simulink model "APE_1"  (R2025a)
settings: Solver=VariableStepAuto  StartTime=0.0  StopTime=1.016  RelTol=1e-3
libraries: spsPWMGeneratorDCDCLib x8, spsCurrentMeasurementLib x5, spsMosfetLib x4, spsSeriesRLCBranchLib x4, spsVoltageMeasurementLib x3, spsDCVoltageSourceLib x1, spsGroundLib x1, eeStairGenerator x1, sps_lib x1
settings Model: Creator=KAILASH  LastModifiedBy=KAILASH

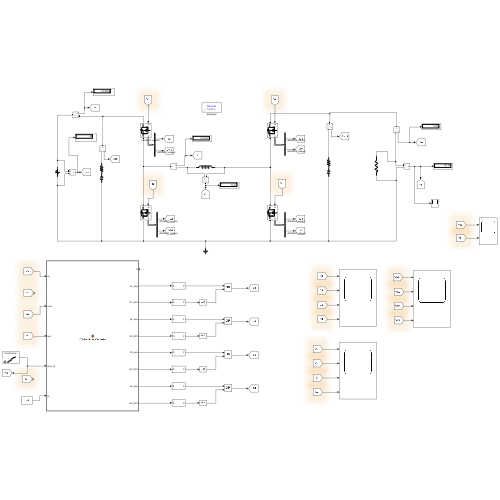
[thumbnail: Simulink's stored preview of the top-level diagram]
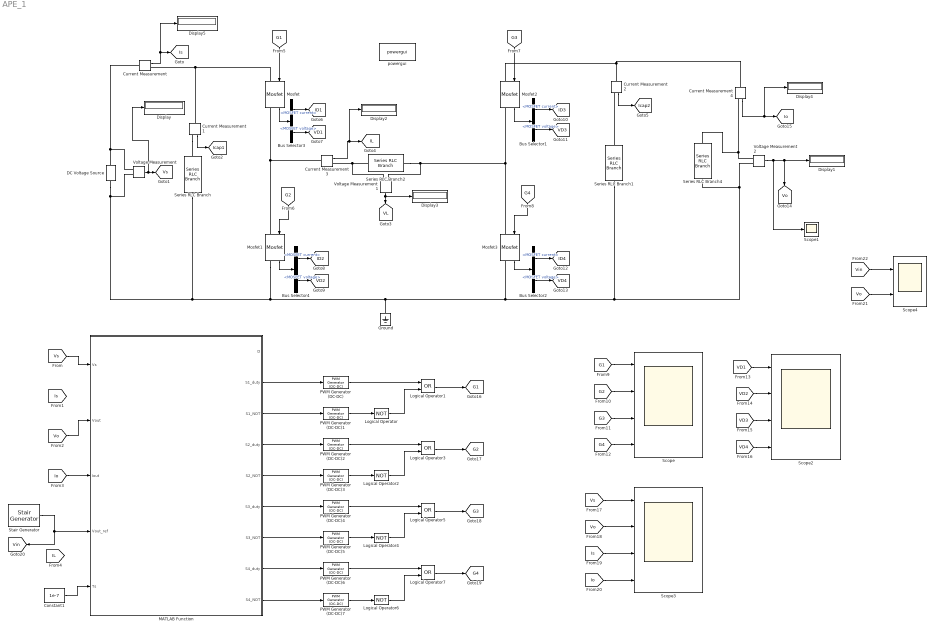
== system APE_1 ==
  Bus Selector{1..4} (4 alike) : BusSelector  OutputSignals=MOSFET current,MOSFET voltage
  Constant1 : Constant  Value=1e-7
  Current Measurement{,1..4} (5 alike) : spsCurrentMeasurementLib/Current Measurement  PhasorSimulation=off  OutputType=Complex  PSBequivalent=0
  DC Voltage Source : spsDCVoltageSourceLib/DC Voltage Source  Amplitude=48  Measurements=Voltage
  Display{,1..5} (6 alike) : Display
  Ground : spsGroundLib/Ground  LConnTagsString=a
  Logical Operator{,2,4,6} (4 alike) : Logic  Operator=NOT  AllPortsSameDT=off  OutDataTypeStr=boolean
  Logical Operator{1,3,5,7} (4 alike) : Logic  Operator=OR  AllPortsSameDT=off  OutDataTypeStr=boolean
  MATLAB Function : MATLAB Function  TreatAsAtomicUnit=on
  Mosfet{,1..3} (4 alike) : spsMosfetLib/Mosfet  Ron=0.01  Lon=0  Rd=0.01  Vfd=0.8  IC=0  Rs=1e5  Cs=inf  Measurements=on
  PWM Generator (DC-DC){,1..7} (8 alike) : spsPWMGeneratorDCDCLib/PWM Generator (DC-DC)  Fsw=75e3  Ts=1e-7
  Scope : Scope  NumInputPorts=4
      settings: ActiveDisplayYMinimum=0.9  ActiveDisplayYMaximum=1.1
  Scope1 : Scope
      settings: ActiveDisplayYMinimum=-11.04407431649155  ActiveDisplayYMaximum=99.45668137748801
  Scope2 : Scope  NumInputPorts=4
      settings: ActiveDisplayYMinimum=-4.0101855999563254  ActiveDisplayYMaximum=36.044750018114769  DataLoggingVariableName=ScopeData2
  Scope3 : Scope  NumInputPorts=4
      settings: ActiveDisplayYMinimum=38  ActiveDisplayYMaximum=58  DataLoggingVariableName=ScopeData3
  Scope4 : Scope  NumInputPorts=2
      settings: ActiveDisplayYMinimum=-26.842242201674949  ActiveDisplayYMaximum=241.58017981507462  DataLoggingVariableName=ScopeData4
  Series RLC Branch : spsSeriesRLCBranchLib/Series RLC Branch  LConnTagsString=__new0  RConnTagsString=__new0  BranchType=RC  Resistance=0.001  Inductance=1e-3  SetiL0=off  InitialCurrent=0  Capacitance=488e-6  Setx0=off  InitialVoltage=48  Measurements=None
  Series RLC Branch1 : spsSeriesRLCBranchLib/Series RLC Branch  LConnTagsString=__new0  RConnTagsString=__new0  BranchType=RC  Resistance=0.01  Inductance=1e-3  SetiL0=off  InitialCurrent=0  Capacitance=488e-6  Setx0=off  InitialVoltage=36  Measurements=None
  Series RLC Branch2 : spsSeriesRLCBranchLib/Series RLC Branch  LConnTagsString=__new0  RConnTagsString=__new0  BranchType=L  Resistance=1  Inductance=150e-6  SetiL0=off  InitialCurrent=0  Capacitance=1e-6  Setx0=off  InitialVoltage=0  Measurements=None
  Series RLC Branch4 : spsSeriesRLCBranchLib/Series RLC Branch  LConnTagsString=__new0  RConnTagsString=__new0  BranchType=R  Resistance=50  Inductance=1e-3  SetiL0=off  InitialCurrent=0  Capacitance=1e-6  Setx0=off  InitialVoltage=0  Measurements=None
  Stair Generator : eeStairGenerator/Stair Generator  LabelModeActiveChoice=Continuous  TimeInput=[0.05 0.4 0.9 1.3 1.7]  AmplitudeInput=[24 36 56 68 80]  SampleTime=0  RepeatPattern=off  OutDataTypeStr=double
      settings: LibrarySourceBlock=ee_sl_lib/General Control/Stair Generator
  Voltage Measurement : spsVoltageMeasurementLib/Voltage Measurement  PhasorSimulation=off  OutputType=Complex  PSBequivalent=0
  Voltage Measurement1 : spsVoltageMeasurementLib/Voltage Measurement  PhasorSimulation=off  OutputType=Complex  PSBequivalent=0
  Voltage Measurement2 : spsVoltageMeasurementLib/Voltage Measurement  PhasorSimulation=off  OutputType=Complex  PSBequivalent=0
  powergui : sps_lib/powergui  Priority=1  SimulationMode=Discrete  SampleTime=1e-7  frequency=60  Iterations=50  frequencyindice=0  Pbase=100e6  ErrMax=1e-4  UnitsV=kV  UnitsW=MW  buscounter=0  FunctionMessages=off  echomessages=off  EnableUseOfTLC=off  CurrentSourceSwitches=off  DisableSnubberDevices=off  DisableRonSwitches=off  DisableVfSwitches=off  DisplayEquations=off  AutomaticDiscreteSolvers=off  SolverType=Tustin/Backward Euler (TBE)  Interpol=off  ExternalGateDelay=off  methode=off  Ts=100  x0status=blocks  SPID=on  SwTol=0  HookPort=off  NonlinearTolerance=1e-4  nMaxIteration=100  ContinueOnMaxIteration=off  RestoreLinks=warning  ResistiveCurrentMeasurement=off  Frange=[0:2:500]  Ylog=off  Xlog=on  ShowGrid=off  save=off  variable=ZData  structure=0  ZoomFFT=off  StartTime=0.0  cycles=1  DisplayStyle=1  fundamental=60  FreqAxis=off  MaxFrequency=1000  frequencyindicesteady=1  RmsSteady=1  display=off
  tag scope: G1=global, G2=global, G3=global, G4=global, ID1=global, ID2=global, ID3=global, ID4=global, IL=global, Icap1=global, Icap2=global, Io=global, Is=global, VD1=global, VD2=global, VD3=global, VD4=global, VL=global, Vin=global, Vo=global, Vs=global
  wires:
  [Is] -> Scope3/3
  MATLAB Function/4(S2_duty) -> PWM Generator (DC-DC)2/1
  PWM Generator (DC-DC)4/1 -> Logical Operator5/1
  [Io] -> Scope3/4
  PWM Generator (DC-DC)/1 -> Logical Operator1/1
  Voltage Measurement1/1 -> Display3/1, [VL]
  Logical Operator6/1 -> Logical Operator7/2
  Logical Operator4/1 -> Logical Operator5/2
  Logical Operator/1 -> Logical Operator1/2
  Current Measurement3/1 -> Display2/1, [IL]
  Current Measurement4/1 -> Display4/1, [Io]
  PWM Generator (DC-DC)2/1 -> Logical Operator3/1
  PWM Generator (DC-DC)7/1 -> Logical Operator6/1
  Bus Selector4/2 -> [VD2]  "<MOSFET voltage>"
  [G2] -> Mosfet1/1
  [G1] -> Mosfet/1
  Bus Selector4/1 -> [ID2]  "<MOSFET current>"
  [Vs] -> Scope3/1
  Mosfet3/1 -> Bus Selector2/1
  MATLAB Function/5(S2_NOT) -> PWM Generator (DC-DC)3/1
  [VD3] -> Scope2/3
  Current Measurement2/1 -> [Icap2]
  Stair Generator/1 -> [Vin], MATLAB Function/4(Vout_ref)
  [G4] -> Mosfet3/1
  Bus Selector2/2 -> [VD4]  "<MOSFET voltage>"
  [G1] -> Scope/1
  Voltage Measurement2/1 -> Scope1/1, [Vo], Display1/1
  MATLAB Function/3(S1_NOT) -> PWM Generator (DC-DC)1/1
  MATLAB Function/9(S4_NOT) -> PWM Generator (DC-DC)7/1
  Bus Selector1/2 -> [VD3]  "<MOSFET voltage>"
  [Vo] -> MATLAB Function/2(Vout)
  Logical Operator7/1 -> [G4]
  [VD2] -> Scope2/2
  [VD4] -> Scope2/4
  Current Measurement1/1 -> [Icap1]
  Current Measurement/1 -> Display5/1, [Is]
  PWM Generator (DC-DC)5/1 -> Logical Operator4/1
  Mosfet1/1 -> Bus Selector4/1
  [G3] -> Scope/3
  Bus Selector2/1 -> [ID4]  "<MOSFET current>"
  PWM Generator (DC-DC)3/1 -> Logical Operator2/1
  Logical Operator5/1 -> [G3]
  [G4] -> Scope/4
  [G2] -> Scope/2
  MATLAB Function/2(S1_duty) -> PWM Generator (DC-DC)/1
  [Io] -> MATLAB Function/3(Iout)
  MATLAB Function/8(S4_duty) -> PWM Generator (DC-DC)6/1
  PWM Generator (DC-DC)6/1 -> Logical Operator7/1
  Bus Selector1/1 -> [ID3]  "<MOSFET current>"
  Constant1/1 -> MATLAB Function/5(Ts)
  Logical Operator3/1 -> [G2]
  [G3] -> Mosfet2/1
  PWM Generator (DC-DC)1/1 -> Logical Operator/1
  Bus Selector3/1 -> [ID1]  "<MOSFET current>"
  [Vo] -> Scope4/2
  Logical Operator2/1 -> Logical Operator3/2
  Logical Operator1/1 -> [G1]
  [VD1] -> Scope2/1
  [Vin] -> Scope4/1
  MATLAB Function/7(S3_NOT) -> PWM Generator (DC-DC)5/1
  [Vo] -> Scope3/2
  Mosfet/1 -> Bus Selector3/1
  MATLAB Function/6(S3_duty) -> PWM Generator (DC-DC)4/1
  Voltage Measurement/1 -> Display/1, [Vs]
  Bus Selector3/2 -> [VD1]  "<MOSFET voltage>"
  Mosfet2/1 -> Bus Selector1/1
  [Vs] -> MATLAB Function/1(Vs)
  connections:
  Series RLC Branch2/RConn1 -- Voltage Measurement1/LConn2 -- Mosfet3/LConn1 -- Mosfet2/RConn1
  DC Voltage Source/LConn1 -- Voltage Measurement/LConn2 -- Mosfet3/RConn1 -- Series RLC Branch1/RConn1 -- Voltage Measurement2/LConn2 -- Series RLC Branch4/RConn1 -- Ground/LConn1 -- Mosfet1/RConn1 -- Series RLC Branch/RConn1
  Mosfet1/LConn1 -- Current Measurement3/LConn1 -- Mosfet/RConn1
  Current Measurement2/LConn1 -- Mosfet2/LConn1 -- Current Measurement4/LConn1
  DC Voltage Source/RConn1 -- Voltage Measurement/LConn1 -- Current Measurement/LConn1
  Voltage Measurement2/LConn1 -- Current Measurement4/RConn1 -- Series RLC Branch4/LConn1
  Mosfet/LConn1 -- Current Measurement1/LConn1 -- Current Measurement/RConn1
  Series RLC Branch2/LConn1 -- Voltage Measurement1/LConn1 -- Current Measurement3/RConn1
  Current Measurement1/RConn1 -- Series RLC Branch/LConn1
  Series RLC Branch1/LConn1 -- Current Measurement2/RConn1

== matlab function APE_1/MATLAB Function ==
  data: Vs input; D output; Vout input; Iout input; Vout_ref input; Ts input; S1_duty output; S1_NOT output; S2_duty output; S2_NOT output; S3_duty output; S3_NOT output; S4_duty output; S4_NOT output
function [D, S1_duty, S1_NOT, S2_duty, S2_NOT, S3_duty, S3_NOT, S4_duty, S4_NOT] = biDirBuckBoostController(Vs, Vout, Iout, Vout_ref, Ts)
% Simplified Bidirectional 4-switch DC-DC controller
% Single Cascaded Loop (Voltage -> Current) with Clamping Anti-Windup
% %#codegen

%% ===================== GLOBAL LIMITS & GAINS =====================
% Duty Cycle Limits (Inner Loop)
D_MAX = 1.0; 
D_MIN = 0.0;
V_HYST = 4.5; % Hysteresis band (V) for topology switching

% Outer Loop (Voltage) Limits & Gains
% NOTE: Set to [5, -5] to prevent the "Inductor Bomb" since you have no Rate Limiter!
I_MAX = 5.0;   
I_MIN = -5.0;  
Kp_v = 0.02;       
Ki_v = 1.0;  

% Inner Loop (Current) Limits & Gains
Kp_i = 0.1;        
Ki_i = 40.0;  

%% ===================== STATE VARIABLES =====================
persistent v_int i_int
if isempty(v_int), v_int = 0; end
if isempty(i_int), i_int = 0; end

%% ===================== OUTER VOLTAGE LOOP (PI 2) =====================
% 1. Calculate Error (Direct from Step input, no Rate Limiter)
v_err = Vout_ref - Vout;

% 2. Calculate P and I terms
v_P = Kp_v * v_err;
v_I_step = Ki_v * v_err * Ts;

% 3. Calculate proposed un-saturated current target
I_unsat = v_P + v_int + v_I_step;

% 4. Clamping Anti-windup (Outer Loop)
if (I_unsat > I_MAX && v_err > 0) || (I_unsat < I_MIN && v_err < 0)
    % Freeze integrator (Do nothing)
else
    v_int = v_int + v_I_step; % Accumulate safe step
end

% 5. Set Final Saturated Current Target
I_target = min(max(v_P + v_int, I_MIN), I_MAX);

%% ===================== INNER CURRENT LOOP (PI 1) =====================
% 1. Calculate Error
i_err = I_target - Iout;

% 2. Calculate P and I terms
i_P = Kp_i * i_err;
i_I_step = Ki_i * i_err * Ts;

% 3. Calculate proposed un-saturated duty cycle
D_unsat = i_P + i_int + i_I_step;

% 4. Clamping Anti-windup (Inner Loop)
if (D_unsat > D_MAX && i_err > 0) || (D_unsat < D_MIN && i_err < 0)
    % Freeze integrator (Do nothing)
else
    i_int = i_int + i_I_step; % Accumulate safe step
end

% 5. Set Final Saturated Duty Cycle
D = min(max(i_P + i_int, D_MIN), D_MAX);

%% ===================== SWITCH MAPPING (TOPOLOGY LOGIC) =====================
if Vs > Vout - V_HYST && Vs < Vout + V_HYST
    % Buck-boost region
    S1_duty = D;      S1_NOT  = 1.0;
    S2_duty = 0.0;    S2_NOT  = D;
    S3_duty = 0.0;    S3_NOT  = D;
    S4_duty = D;      S4_NOT  = 1.0;
elseif Vs > Vout + V_HYST
    % Buck region
    S1_duty = D;      S1_NOT  = 1.0;
    S2_duty = 0.0;    S2_NOT  = D;
    S3_duty = 1.0;    S3_NOT  = 1.0;
    S4_duty = 0.0;    S4_NOT  = 1.0;
else
    % Boost region 
    S1_duty = 1.0;    S1_NOT  = 1.0;
    S2_duty = 0.0;    S2_NOT  = 1.0;
    S3_duty = 0.0;    S3_NOT  = D;
    S4_duty = D;      S4_NOT  = 1.0;
end

end
